simulink library "bsd"  (Simulink 8.1)
settings: Solver=ode1  StartTime=0.0  StopTime=Inf  FixedStep=0.001  RelTol=1e-3
PostLoadFcn:
  | , if any(exist('dsrtsu_mdlpostloadfcn', 'file') == [2, 3, 6]), try dsrtsu_mdlpostloadfcn('Execute', bdroot); catch fprintf('Error in PostLoadFcn (dsrtsu_mdlpostloadfcn) for model "%s":\n %s\n', bdroot, lasterr); end, end,
undefined symbols (not defined in the file or in its folder): KACC_ACCBrakeDisableSpd_kph, KACC_SteadyDistControlDesDist_m, KACC_SteadyDistControlPerc_perc, KACC_SteadyDistCtrlPTBFixedMarg_flg
libraries: hcu_lib x1
settings Model: DSRTSU_INTERNAL_RTI_VER=450  DSRTSU_INTERNAL_RTI_TYPE=rti1401  Creator=AT015555  LastModifiedBy=AT015555

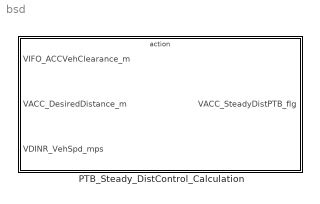
== system bsd ==
  PTB_Steady_DistControl_Calculation : Subsystem  TreatAsAtomicUnit=on

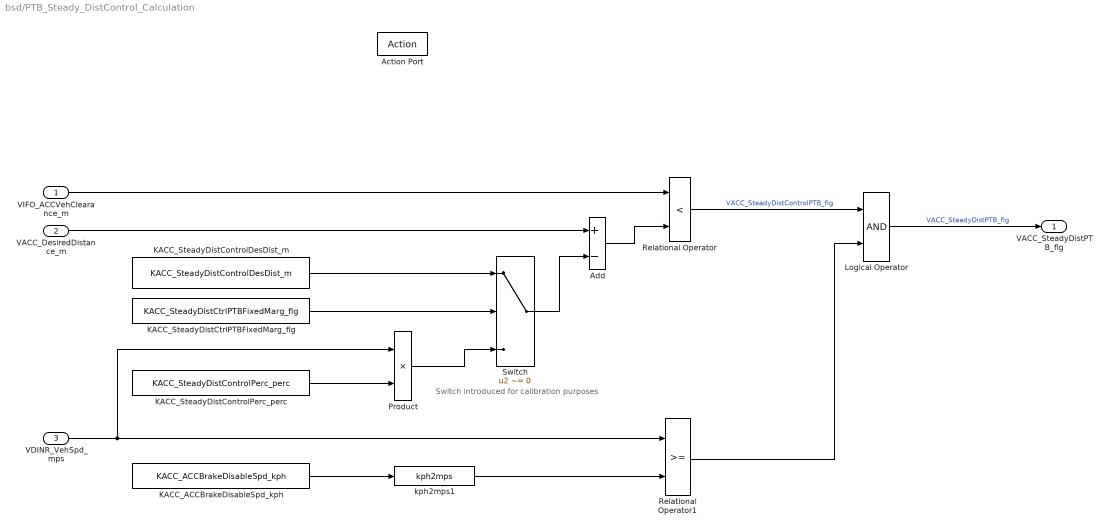
== system bsd/PTB_Steady_DistControl_Calculation ==
  note: Switch introduced for calibration purposes
  VIFO_ACCVehClearance_m : Inport
  VACC_DesiredDistance_m : Inport  Port=2
  VDINR_VehSpd_mps : Inport  Port=3
  Action Port : ActionPort
  Add : Sum  Inputs=+-
  KACC_ACCBrakeDisableSpd_kph : Constant  Value=KACC_ACCBrakeDisableSpd_kph
  KACC_SteadyDistControlDesDist_m : Constant  Value=KACC_SteadyDistControlDesDist_m
  KACC_SteadyDistControlPerc_perc : Constant  Value=KACC_SteadyDistControlPerc_perc
  KACC_SteadyDistCtrlPTBFixedMarg_flg : Constant  Value=KACC_SteadyDistCtrlPTBFixedMarg_flg
  Logical Operator : Logic  AllPortsSameDT=off  OutDataTypeStr=boolean
  Product : Product
  Relational Operator : RelationalOperator  Operator=<  OutDataTypeStr=boolean
  Relational Operator1 : RelationalOperator  OutDataTypeStr=boolean
  Switch : Switch  Criteria=u2 ~= 0
  kph2mps1 : hcu_lib/kph2mps
  VACC_SteadyDistPTB_flg : Outport
  wires:
  Relational Operator1/1 -> Logical Operator/2
  Relational Operator/1 -> Logical Operator/1  "VACC_SteadyDistControlPTB_flg"
  KACC_ACCBrakeDisableSpd_kph/1 -> kph2mps1/1
  Logical Operator/1 -> VACC_SteadyDistPTB_flg/1  "VACC_SteadyDistPTB_flg"
  VACC_DesiredDistance_m/1 -> Add/1
  Add/1 -> Relational Operator/2
  VIFO_ACCVehClearance_m/1 -> Relational Operator/1
  VDINR_VehSpd_mps/1 -> Relational Operator1/1, Product/1
  KACC_SteadyDistCtrlPTBFixedMarg_flg/1 -> Switch/2
  KACC_SteadyDistControlPerc_perc/1 -> Product/2
  Product/1 -> Switch/3
  Switch/1 -> Add/2
  KACC_SteadyDistControlDesDist_m/1 -> Switch/1
  kph2mps1/1 -> Relational Operator1/2
